simulink model "q1_model"  (R2021b)
settings: Solver=FixedStepAuto  StartTime=0.0  StopTime=0.2  FixedStep=dt  RelTol=1e-3
values from neighbouring files (symbols this model uses):
  CLVD = .0146    (= 0.0146)    [Q1_init.m]
  CLVS = .00003    (= 3e-05)    [Q1_init.m]
  Csa = .00175    (= 0.00175)    [Q1_init.m]
  Pla = 5    [Q1_init.m]
  Plvi = 5    [Q1_init.m]
  Psai = 80    [Q1_init.m]
  RAo = .01    (= 0.01)    [Q1_init.m]
  Rmi = .01    (= 0.01)    [Q1_init.m]
  Rs = 17.86    [Q1_init.m]
  T = 0.0125    [Q1_init.m]
  tauD = .001    (= 0.001)    [Q1_init.m]
  tauS = .0025    (= 0.0025)    [Q1_init.m]
  Ts = 0.0050    (= 0.005)    [Q1_init.m]
settings Model: Creator=jeff  LastModifiedBy=jeff

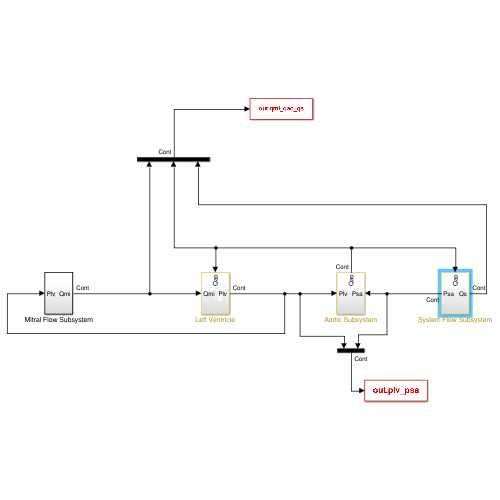
[thumbnail: Simulink's stored preview of the top-level diagram]
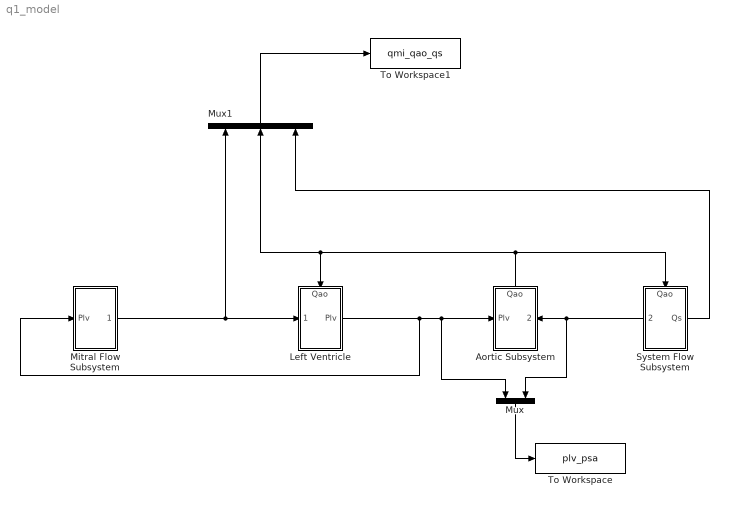
== system q1_model ==
  Aortic Subsystem : Subsystem
      settings: PortSchema="{\"entries\":[{\"content\":{\"sides\":[{\"content\":{\"connectorIds\":[\"In1\"]},\"type\":\"ConnectorPlacement.EquallySpacedRectSide\",\"uuid\":\"9d62a5ea-3505-45d4-b119-238d7ae834df\"},{\"content\":{\"connectorIds\":[\"In2\"],\"side\":\"RIGHT\"},\"type\":\"ConnectorPlacement.EquallySpacedRectSide\",\"uuid\":\"0c5e2ede-72a3-4098-af13-c35576c08d5e\"},{\"content\":{\"connectorIds\":[\"Out1\"],\"side\":\"TOP\"},\"type\":\"ConnectorPlacement.EquallySpacedRectSide\",\"uuid\":\"96cf0109-cc5d-4267-af88-21999f5ed5c2\"},{\"content\":{\"connectorIds\":[],\"side\":\"BOTTOM\"},\"type\":\"ConnectorPlacement.EquallySpacedRectSide\",\"uuid\":\"c3f6794c-2e65-4a32-adad-4e5f02023522\"}]},\"type\":\"ConnectorPlacement.EquallySpacedConnector\",\"uuid\":\"045e0f28-3cf5-4e8b-83f1-350fdf43b46e\"}],\"packageUris\":[\"http://schema.mathworks.com/mf0/Connector/R2020b\"],\"version\":\"1.0\"}"
  Left Ventricle : Subsystem
      settings: PortSchema="{\"entries\":[{\"content\":{\"sides\":[{\"content\":{\"connectorIds\":[\"In1\"]},\"type\":\"ConnectorPlacement.EquallySpacedRectSide\",\"uuid\":\"9d62a5ea-3505-45d4-b119-238d7ae834df\"},{\"content\":{\"connectorIds\":[\"Out1\"],\"side\":\"RIGHT\"},\"type\":\"ConnectorPlacement.EquallySpacedRectSide\",\"uuid\":\"0c5e2ede-72a3-4098-af13-c35576c08d5e\"},{\"content\":{\"connectorIds\":[\"In2\"],\"side\":\"TOP\"},\"type\":\"ConnectorPlacement.EquallySpacedRectSide\",\"uuid\":\"96cf0109-cc5d-4267-af88-21999f5ed5c2\"},{\"content\":{\"connectorIds\":[],\"side\":\"BOTTOM\"},\"type\":\"ConnectorPlacement.EquallySpacedRectSide\",\"uuid\":\"cbda366c-c898-4ae7-a133-3dc5c5c3fc73\"}]},\"type\":\"ConnectorPlacement.EquallySpacedConnector\",\"uuid\":\"045e0f28-3cf5-4e8b-83f1-350fdf43b46e\"}],\"packageUris\":[\"http://schema.mathworks.com/mf0/Connector/R2020b\"],\"version\":\"1.0\"}"
  Mitral Flow Subsystem : Subsystem
  Mux : Mux  Inputs=2
  Mux1 : Mux  Inputs=3
  System Flow Subsystem : Subsystem
      settings: PortSchema="{\"entries\":[{\"content\":{\"sides\":[{\"content\":{\"connectorIds\":[\"Out2\"]},\"type\":\"ConnectorPlacement.EquallySpacedRectSide\",\"uuid\":\"4fa4a1e0-8a26-47a7-8728-447bee4a4971\"},{\"content\":{\"connectorIds\":[\"Out1\"],\"side\":\"RIGHT\"},\"type\":\"ConnectorPlacement.EquallySpacedRectSide\",\"uuid\":\"09528f8c-f905-4103-939c-a6d150bb3e04\"},{\"content\":{\"connectorIds\":[\"In1\"],\"side\":\"TOP\"},\"type\":\"ConnectorPlacement.EquallySpacedRectSide\",\"uuid\":\"6ed22675-0162-4d6d-bd7b-89e8d30e014c\"}]},\"type\":\"ConnectorPlacement.EquallySpacedConnector\",\"uuid\":\"c610c103-1d04-417b-80da-fcbf8cfee0c6\"}],\"packageUris\":[\"http://schema.mathworks.com/mf0/Connector/R2020b\"],\"version\":\"1.0\"}"
  To Workspace : ToWorkspace  VariableName=plv_psa  SaveFormat=Timeseries  SampleTime=-1
  To Workspace1 : ToWorkspace  VariableName=qmi_qao_qs  SaveFormat=Timeseries  SampleTime=-1
  wires:
  Aortic Subsystem/1(Qao) -> System Flow Subsystem/1(Qao), Mux1/2, Left Ventricle/2(Qao)
  Mitral Flow Subsystem/1(Qmi) -> Mux1/1, Left Ventricle/1(Qmi)
  System Flow Subsystem/1(Qs) -> Mux1/3
  Left Ventricle/1(Plv) -> Mitral Flow Subsystem/1(Plv), Mux/1, Aortic Subsystem/1(Plv)
  System Flow Subsystem/2(Psa) -> Mux/2, Aortic Subsystem/2(Psa)
  Mux/1 -> To Workspace/1
  Mux1/1 -> To Workspace1/1

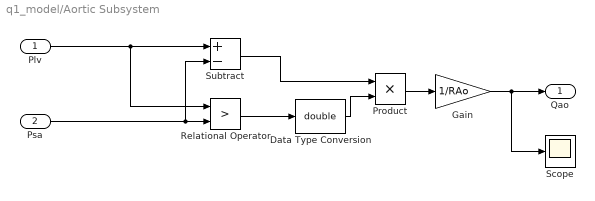
== system q1_model/Aortic Subsystem ==
  Plv : Inport
  Psa : Inport  Port=2
  Data Type Conversion : DataTypeConversion  OutDataTypeStr=double
  Gain : Gain  Gain=1/RAo
  Product : Product  RndMeth=Zero
  Relational Operator : RelationalOperator  Operator=>  OutDataTypeStr=boolean  RndMeth=Nearest
  Scope : Scope
  Subtract : Sum  Inputs=+-
  Qao : Outport
  wires:
  Data Type Conversion/1 -> Product/2
  Subtract/1 -> Product/1
  Product/1 -> Gain/1
  Relational Operator/1 -> Data Type Conversion/1
  Gain/1 -> Scope/1, Qao/1
  Plv/1 -> Subtract/1, Relational Operator/1
  Psa/1 -> Subtract/2, Relational Operator/2

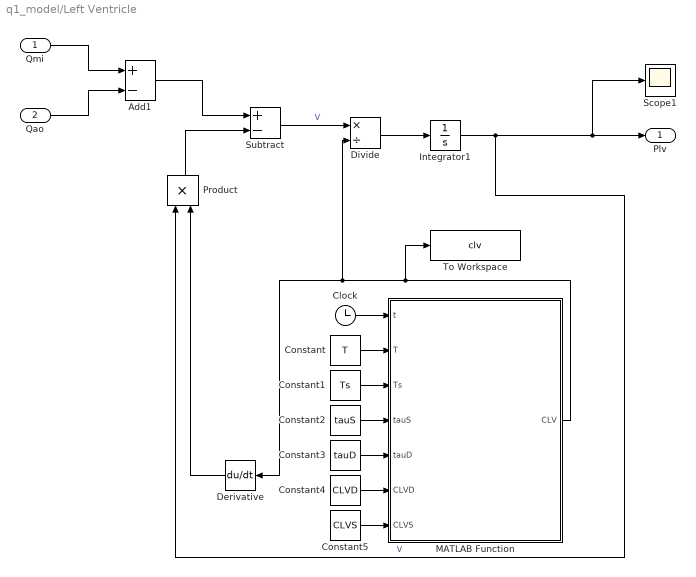
== system q1_model/Left Ventricle ==
  Qmi : Inport
  Qao : Inport  Port=2
  Add1 : Sum  Inputs=+-
  Clock : Clock
  Constant : Constant  Value=T
  Constant1 : Constant  Value=Ts
  Constant2 : Constant  Value=tauS
  Constant3 : Constant  Value=tauD
  Constant4 : Constant  Value=CLVD
  Constant5 : Constant  Value=CLVS
  Derivative : Derivative
  Divide : Product  Inputs=*/
  Integrator1 : Integrator  InitialCondition=Plvi
  MATLAB Function : MATLAB Function  TreatAsAtomicUnit=on
  Product : Product
  Scope1 : Scope
  Subtract : Sum  Inputs=+-
  To Workspace : ToWorkspace  VariableName=clv  SaveFormat=Timeseries  SampleTime=-1
  Plv : Outport
  wires:
  Qao/1 -> Add1/2
  Qmi/1 -> Add1/1
  Clock/1 -> MATLAB Function/1(t)
  Subtract/1 -> Divide/1  "V"
  Constant/1 -> MATLAB Function/2(T)
  Constant1/1 -> MATLAB Function/3(Ts)
  Constant2/1 -> MATLAB Function/4(tauS)
  Constant3/1 -> MATLAB Function/5(tauD)
  Constant4/1 -> MATLAB Function/6(CLVD)
  Constant5/1 -> MATLAB Function/7(CLVS)
  Add1/1 -> Subtract/1
  MATLAB Function/1(CLV) -> To Workspace/1, Derivative/1, Divide/2
  Product/1 -> Subtract/2
  Integrator1/1 -> Plv/1, Scope1/1, Product/1  "V"
  Divide/1 -> Integrator1/1
  Derivative/1 -> Product/2

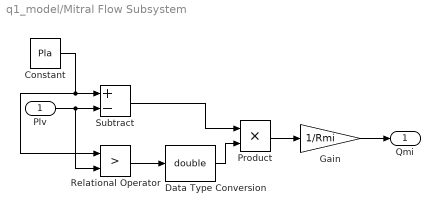
== system q1_model/Mitral Flow Subsystem ==
  Plv : Inport
  Constant : Constant  Value=Pla
  Data Type Conversion : DataTypeConversion  OutDataTypeStr=double
  Gain : Gain  Gain=1/Rmi
  Product : Product  RndMeth=Zero
  Relational Operator : RelationalOperator  Operator=>  OutDataTypeStr=boolean  RndMeth=Nearest
  Subtract : Sum  Inputs=+-
  Qmi : Outport
  wires:
  Product/1 -> Gain/1
  Relational Operator/1 -> Data Type Conversion/1
  Plv/1 -> Relational Operator/2, Subtract/2
  Data Type Conversion/1 -> Product/2
  Subtract/1 -> Product/1
  Constant/1 -> Relational Operator/1, Subtract/1
  Gain/1 -> Qmi/1

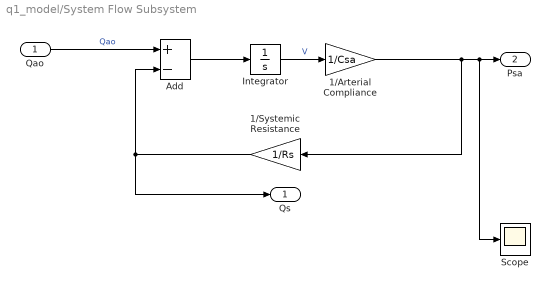
== system q1_model/System Flow Subsystem ==
  Qao : Inport
  1/Arterial Compliance : Gain  Gain=1/Csa
  "1/Systemic Resistance " : Gain  Gain=1/Rs
  Add : Sum  Inputs=+-
  Integrator : Integrator  InitialCondition=Psai*Csa
  Scope : Scope
  Qs : Outport
  Psa : Outport  Port=2
  wires:
  Integrator/1 -> 1/Arterial Compliance/1  "V"
  Qao/1 -> Add/1  "Qao"
  "1/Systemic Resistance "/1 -> Qs/1, Add/2
  Add/1 -> Integrator/1
  1/Arterial Compliance/1 -> "1/Systemic Resistance "/1, Scope/1, Psa/1

== matlab function q1_model/Left Ventricle/MATLAB Function ==
  data: t input; CLV output; T input; Ts input; tauS input; tauD input; CLVD input; CLVS input
function CLV=CLV_now(t, T, Ts, tauS, tauD, CLVD, CLVS) 
tc=rem(t,T); 
%tc=time in the current cycle, 
%measured  from  start  of systole. 
if(tc<Ts) 
    e=(1-exp(-tc/tauS))/(1-exp(-Ts/tauS)); 
    CLV=CLVD*(CLVS/CLVD)^e; 
else 
    e=(1-exp(-(tc-Ts)/tauD))/(1-exp(-(T-Ts)/tauD)); 
    CLV=CLVS*(CLVD/CLVS)^e; 
end
